simulink model "closedloop_PI"  (R2022b)
settings: Solver=ode15s  StartTime=0.0  StopTime=75  RelTol=1e-7  AbsTol=1e-7  EnableMultiTasking=on
InitFcn:
  | datacstr
undefined symbols (not defined in the file or in its folder): c_bar, cf_bar, cp, cstrfun, DH, ER, ko, Kpp, q, r, T_bar, Tc_bar, Tf, UA, V
settings Model: Creator=scattolini  LastModifiedBy=marco
settings SolverCC: AutoScaleAbsTol=off  AlgebraicLoopSolver=TrustRegion
settings DataIOCC: SaveFormat=Array  SignalLoggingSaveFormat=ModelDataLogs  ReturnWorkspaceOutputs=off  SignalLoggingName=sigsOut
settings OptimizationCC: BlockReduction=off  BooleanDataType=off  DefaultParameterBehavior=Inlined  BufferReuse=off  ExpressionDepthLimit=2147483647  InitFltsAndDblsToZero=on  LifeSpan=inf
settings DebuggingCC: SaveWithParameterizedLinksMsg=none  UnderspecifiedInitializationDetection=Classic  MergeDetectMultiDrivingBlocksExec=none  SignalResolutionControl=TryResolveAllWithWarning  MultiTaskDSMMsg=warning  MultiTaskCondExecSysMsg=none  FcnCallInpInsideContextMsg=warning  UnconnectedInputMsg=warning  UnconnectedOutputMsg=warning  UnconnectedLineMsg=warning  StateNameClashWarn=warning  SFUnexpectedBacktrackingDiag=warning  SFNoUnconditionalDefaultTransitionDiag=warning  SFExecutionAtInitializationDiag=none  SFMachineParentedDataDiag=warning  ArithmeticOperatorsInVariantConditions=warning
settings HardwareCC: ProdBitPerPointer=32  ProdBitPerSizeT=32  ProdBitPerPtrDiffT=32  ProdLargestAtomicFloat=None  ProdIntDivRoundTo=Undefined  ProdEndianess=Unspecified  ProdWordSize=32  ProdHWDeviceType=32-bit Generic  TargetUnknown=on
settings ModelReferenceCC: EnableRefExpFcnMdlSchedulingChecks=on  PropagateSignalLabelsOutOfModel=off
settings SFSimCC: SimUseLocalCustomCode=off  CustomCodeUndefinedFunction=UseInterfaceOnly
settings RTWCC: RTWUseLocalCustomCode=off  DLArmComputeVersion=19.05
settings CodeAppCC: StateflowObjectComments=on
settings GRTTargetCC: TargetFcnLib=ansi_tfl_tmw.mat  TargetLangStandard=C89/C90 (ANSI)  CombineOutputUpdateFcns=off  GRTInterface=on
settings ConfigComp: CovMetricSettings=dw  CovSaveCumulativeToWorkspaceVar=on  CovSaveSingleToWorkspaceVar=on  CovExternalEMLEnable=off  CovSFcnEnable=off

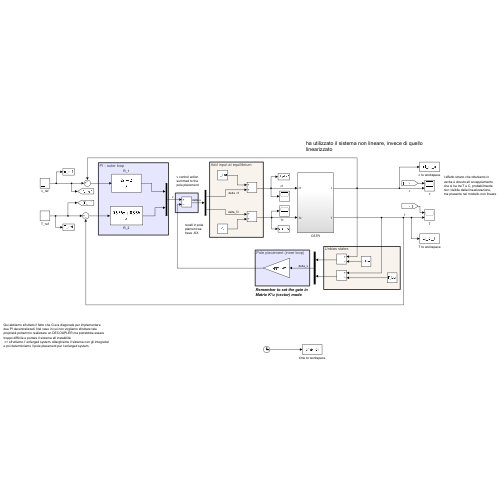
[thumbnail: Simulink's stored preview of the top-level diagram]
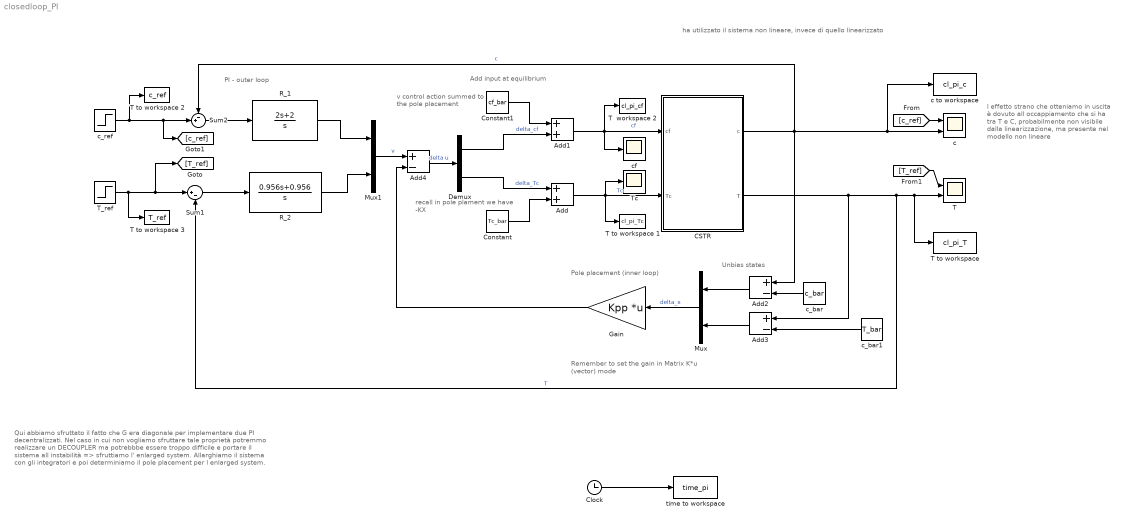
== system closedloop_PI ==
  note: Qui abbiamo sfruttato il fatto che G era diagonale per implementare
      | due PI decentralizzati. Nel caso in cui non vogliamo sfruttare tale
      | proprietà potremmo realizzare un DECOUPLER ma potrebbbe essere
      | troppo difficile e portare il sistema all instabilità
      |  => sfruttiamo l' enlarged system. Allarghiamo il sistema con gli integratori
      | e poi determiniamo il pole placement per l enlarged system.
  note: l effetto strano che otteniamo in
      | uscita è dovuto all occappiamento
      | che si ha tra T e C, probabilmente
      | non visibile dalla linearizzazione,
      | ma presente nel modello non lineare
  note: recall in pole
      | plament we
      | have -KX
  note: v control action
      | summed to the
      | pole placement
  note: ha utilizzato il sistema non lineare, invece di quello linearizzato
  note: Unbias states
  note: Add input at equilibrium
  note: Pole placement (inner loop)
  note: PI - outer loop
  note: Remember to set the gain in
      | Matrix K*u (vector) mode
  Add : Sum
  Add1 : Sum
  Add2 : Sum  Inputs=+-
  Add3 : Sum  Inputs=+-
  Add4 : Sum  Inputs=+-
  CSTR : Subsystem
  Clock : Clock
  Constant : Constant  Value=Tc_bar
  Constant1 : Constant  Value=cf_bar
  Demux : Demux  Outputs=2
  Gain : Gain  Gain=Kpp  Multiplication=Matrix(K*u) (u vector)
  Mux : Mux  Inputs=2
  Mux1 : Mux  Inputs=2
  R_1 : TransferFcn  Numerator=[2 2]  Denominator=[1 0]
  R_2 : TransferFcn  Numerator=[0.956, 0.956]  Denominator=[1 0]
  Sum1 : Sum  Inputs=|+-
  Sum2 : Sum  Inputs=-+|
  T : Scope  NumInputPorts=2
  T  workspace 2 : ToWorkspace  VariableName=cl_pi_cf  SampleTime=-1
  "T to workspace " : ToWorkspace  VariableName=cl_pi_T  SampleTime=-1
  T to workspace 1 : ToWorkspace  VariableName=cl_pi_Tc  SampleTime=-1
  T to workspace 2 : ToWorkspace  VariableName=c_ref  SampleTime=-1
  T to workspace 3 : ToWorkspace  VariableName=T_ref  SampleTime=-1
  T_ref : Step  Time=30  Before=350  After=340  SampleTime=0
  Tc : Scope
  c : Scope  NumInputPorts=2
  "c to workspace " : ToWorkspace  VariableName=cl_pi_c  SampleTime=-1
  c_bar : Constant  Value=c_bar
  c_bar1 : Constant  Value=T_bar
  c_ref : Step  Time=10  Before=0.5  After=0.55  SampleTime=0
  cf : Scope
  time to workspace : ToWorkspace  VariableName=time_pi  SampleTime=-1
  wires:
  Clock/1 -> time to workspace/1
  CSTR/1(c) -> Add2/1, c/2, "c to workspace "/1, Sum2/1  "c"
  Add/1 -> Tc/1, T to workspace 1/1, CSTR/2(Tc)  "Tc"
  Constant/1 -> Add/2
  Constant1/1 -> Add1/1
  c_bar/1 -> Add2/2
  c_bar1/1 -> Add3/2
  Add3/1 -> Mux/2
  Add2/1 -> Mux/1
  Mux/1 -> Gain/1  "delta_x"
  Demux/1 -> Add1/2  "delta_cf"
  Demux/2 -> Add/1  "delta_Tc"
  R_1/1 -> Mux1/1
  R_2/1 -> Mux1/2
  Sum1/1 -> R_2/1
  Sum2/1 -> R_1/1
  c_ref/1 -> T to workspace 2/1, [c_ref], Sum2/2
  T_ref/1 -> T to workspace 3/1, [T_ref], Sum1/1
  Gain/1 -> Add4/2
  Add4/1 -> Demux/1  "delta u"
  CSTR/2(T) -> Add3/1, T/2, "T to workspace "/1, Sum1/2  "T"
  Mux1/1 -> Add4/1  "v"
  [c_ref] -> c/1
  [T_ref] -> T/1
  Add1/1 -> cf/1, CSTR/1(cf), T  workspace 2/1  "cf"

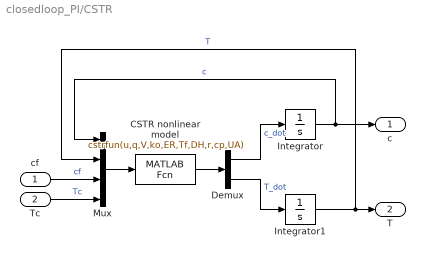
== system closedloop_PI/CSTR ==
  cf : Inport  PortDimensions=1
  Tc : Inport  Port=2  PortDimensions=1
  CSTR nonlinear model : MATLABFcn  MATLABFcn=cstrfun(u,q,V,ko,ER,Tf,DH,r,cp,UA)  OutputDimensions=2
  Demux : Demux  Outputs=2
      settings: DisplayOption=none
  Integrator : Integrator  InitialCondition=c_bar + 0.025
  Integrator1 : Integrator  InitialCondition=T_bar + 2.5
  Mux : Mux
  c : Outport  PortDimensions=1
  T : Outport  Port=2  PortDimensions=1
  wires:
  Mux/1 -> CSTR nonlinear model/1
  CSTR nonlinear model/1 -> Demux/1
  Demux/1 -> Integrator/1  "c_dot"
  Demux/2 -> Integrator1/1  "T_dot"
  Integrator1/1 -> Mux/2, T/1  "T"
  Integrator/1 -> Mux/1, c/1  "c"
  cf/1 -> Mux/3  "cf"
  Tc/1 -> Mux/4  "Tc"
